simulink model "model"  (Simulink 7.8)
settings: Solver=ode45  StartTime=0.0  StopTime=inf  RelTol=1e-3
values from neighbouring files (symbols this model uses):
  q = [x;y;z;a;b;c;theta_W_R;u_W_R;theta_W_L;u_W_L;u_R_R;x_R_R;u_R_L;x_R_L;]    [environment.m]    (also in main_kalker.m = q + delta_q)
settings Model: Creator=imac  LastModifiedBy=aitor
settings DebuggingCC: FcnCallInpInsideContextMsg=Use local settings

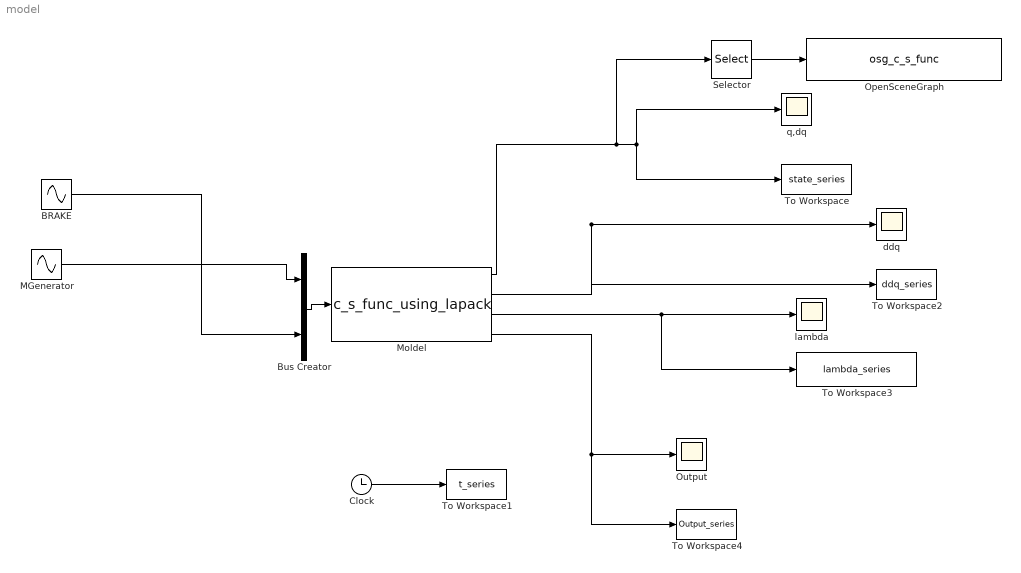
== system model ==
  BRAKE : Sin  Amplitude=0  Frequency=0  Phase=pi/2  SampleTime=0
  Bus Creator : BusCreator  Inputs=2
  Clock : Clock
  MGenerator : Sin  Amplitude=0  Frequency=0  Phase=pi/2  SampleTime=0
  Moldel : S-Function  FunctionName=c_s_func_using_lapack  Parameters=q dq param  EnableBusSupport=off
      mask Type: S-function: mycsfunc
      mask Description: This is a S-function that does the continuous state space system.
      mask Display: disp('[M , Phi_q''] [ddq]\n[Phi_q , 0] [lambda]\n=\n [Q ] \n   [gamma] ');
  OpenSceneGraph : S-Function  FunctionName=osg_c_s_func  EnableBusSupport=off
  Output : Scope
      settings: YMin=0  YMax=1300  SaveName=ScopeData3  SampleInput=on  SampleTime=0.01
  Selector : Selector  InputPortWidth=2*length(q)  IndexOptions=Index vector (dialog)  Indices=1:1:length(q)  OutputSizes=1
  To Workspace : ToWorkspace  VariableName=state_series  SampleTime=0.01  SaveFormat=Array
  To Workspace1 : ToWorkspace  VariableName=t_series  SampleTime=0.01  SaveFormat=Array
  To Workspace2 : ToWorkspace  VariableName=ddq_series  SampleTime=0.01  SaveFormat=Array
  To Workspace3 : ToWorkspace  VariableName=lambda_series  SampleTime=0.01  SaveFormat=Array
  To Workspace4 : ToWorkspace  VariableName=Output_series  SampleTime=0.01  SaveFormat=Array
  ddq : Scope
      settings: YMin=-500  YMax=300  SampleInput=on  SampleTime=0.01
  lambda : Scope
      settings: YMin=-1750  YMax=1000  SaveName=ScopeData2  SampleInput=on  SampleTime=0.01
  q,dq : Scope
      settings: YMin=-0.035  YMax=0.045  SampleInput=on  SampleTime=0.01
  wires:
  Clock/1 -> To Workspace1/1
  Moldel/1 -> q,dq/1, To Workspace/1, Selector/1
  Moldel/2 -> ddq/1, To Workspace2/1
  Moldel/3 -> lambda/1, To Workspace3/1
  Moldel/4 -> Output/1, To Workspace4/1
  Selector/1 -> OpenSceneGraph/1
  Bus Creator/1 -> Moldel/1
  BRAKE/1 -> Bus Creator/2
  MGenerator/1 -> Bus Creator/1
